simulink model "Ctrl_warning"  (R2018b)
settings: Solver=FixedStepDiscrete  StartTime=0.0  StopTime=10.0  FixedStep=0.1  RelTol=1e-3  EnableMultiTasking=on
values from neighbouring files (symbols this model uses):
  BASE_DATA_TYPE = mpt.Parameter    [warnings_interface_dd.m]
  EXTD_PAYLOAD_AVBLSTS = mpt.Parameter    [warnings_interface_dd.m]
  MASTER_LAMP_MASK = mpt.Parameter    [warnings_interface_dd.m]
  RED = mpt.Parameter    [warnings_interface_dd.m]
  WARN_ATTRIBUTES_ARRAY = mpt.Parameter    [Ctrl_warning_config.m]
  WARN_LAMP_CONFIGURED = mpt.Parameter    [Ctrl_warning_config.m]
  WRN_PAYLOAD_INITVAL = mpt.Parameter    [warnings_interface_dd.m]
  YELLOW = mpt.Parameter    [warnings_interface_dd.m]
undefined symbols (not defined in the file or in its folder): ExtWarningCurrentEvent, ExtWarningCurrentPayload, ExtWarningCurrentStatus, TotalNumOfWarnings, UI_WARNING_EVENT_FORCED, UI_WARNING_EVENT_NONE, UI_WARNING_EVENT_RETRIGGER, UI_WARNING_STATUS_OFF, UI_WARNING_STATUS_ON, WRNG_NOTIFIED_NONE, WRNG_NOTIFIED_SHOW
libraries: simulink x31, hdlsllib x3
settings Model: Creator=VRK  LastModifiedBy=VRK
settings DataIOCC: SaveOutput=off
settings OptimizationCC: DefaultParameterBehavior=Inlined  EnhancedBackFolding=on  PassReuseOutputArgsAs=Individual arguments  ZeroExternalMemoryAtStartup=off  ZeroInternalMemoryAtStartup=off  MaxStackSize=750  OptimizeBlockOrder=speed  DifferentSizesBufferReuse=on  OptimizationCustomize=off
settings DebuggingCC: ParameterTunabilityLossMsg=error
settings SFSimCC: MATLABDynamicMemAlloc=off
settings RTWCC: SystemTargetFile=autosar.tlc  GenCodeOnly=on  TemplateMakefile=ert_default_tmf  Description=AUTOSAR  GenerateReport=on  IncludeHyperlinkInReport=on  LaunchReport=on  PortableWordSizes=on  GenerateTraceInfo=on  GenerateTraceReport=on  GenerateTraceReportSl=on  GenerateTraceReportSf=on  GenerateTraceReportEml=on
settings CodeAppCC: ForceParamTrailComments=on  IgnoreCustomStorageClasses=off  OperatorAnnotations=on  SimulinkDataObjDesc=on  SFDataObjDesc=on  InsertBlockDesc=on
settings STFCustomTargetCC: TargetLangStandard=C99 (ISO)  MultiwordLength=256  ParMdlRefBuildCompliant=on  CompOptLevelCompliant=on  IncludeMdlTerminateFcn=off  CombineOutputUpdateFcns=on  SuppressErrorStatus=on  ERTCustomFileBanners=on  SupportNonFinite=off  SupportComplex=off  SupportContinuousTime=off  SupportNonInlinedSFcns=off  RemoveResetFunc=on  ParenthesesLevel=Maximum  CastingMode=Standards  MATLABClassNameForMDSCustomization=Simulink.SoftwareTarget.ERTCustomization  AutosarCompliant=on  UseToolchainInfoCompliant=on  LookupTableObjectStructAxisOrder=2,1,3,4,...  LUTObjectStructOrderEvenSpacing=Size,Table,Breakpoints  SystemTargetFile=autosar.tlc
settings ERTTargetCC: TargetLangStandard=C99 (ISO)  ConcurrentExecutionCompliant=off  IncludeMdlTerminateFcn=off  SuppressErrorStatus=on  SupportNonFinite=off  SupportComplex=off  ParenthesesLevel=Maximum  CastingMode=Standards  ModelStepFunctionPrototypeControlCompliant=off  CPPClassGenCompliant=off  AutosarCompliant=on  LookupTableObjectStructAxisOrder=2,1,3,4,...  LUTObjectStructOrderEvenSpacing=Size,Table,Breakpoints  InlinedParameterPlacement=NonHierarchical  ERTCustomFileTemplate=example_file_process.tlc  ERTFilePackagingFormat=CompactWithDataFile

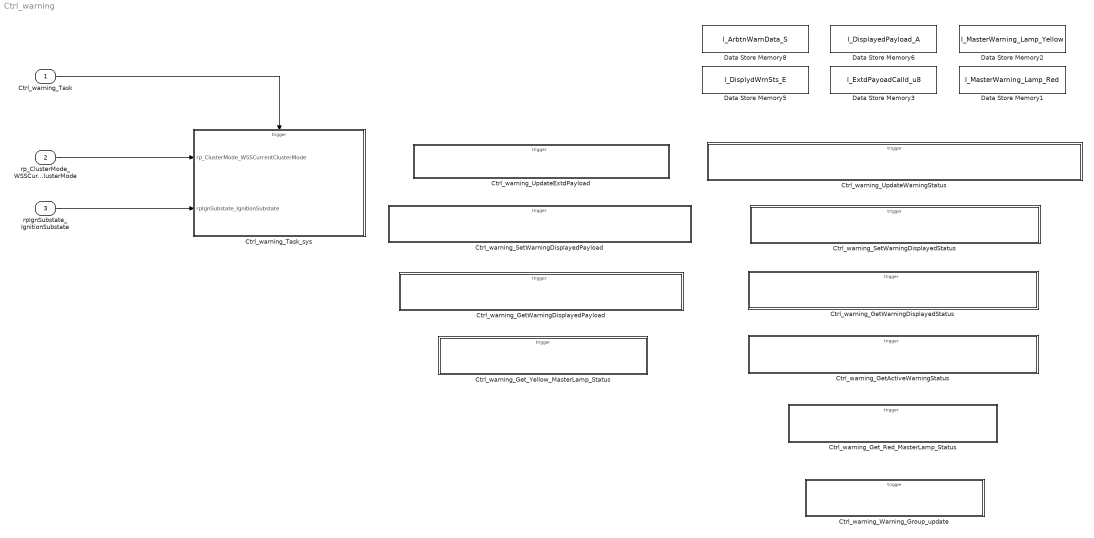
== system Ctrl_warning ==
  Ctrl_warning_Task : Inport  SampleTime=0.1  OutputFunctionCall=on
  rp_ClusterMode_WSSCurrentClusterMode : Inport  Port=2  OutDataTypeStr=ClusterModes  PortDimensions=1
  rpIgnSubstate_IgnitionSubstate : Inport  Port=3  OutDataTypeStr=IgntionSubstateType  PortDimensions=1
  Ctrl_warning_GetActiveWarningStatus : Subsystem  TreatAsAtomicUnit=on
  Ctrl_warning_GetWarningDisplayedPayload : Subsystem  TreatAsAtomicUnit=on
  Ctrl_warning_GetWarningDisplayedStatus : Subsystem  TreatAsAtomicUnit=on
  Ctrl_warning_Get_Red_MasterLamp_Status : Subsystem  TreatAsAtomicUnit=on
  Ctrl_warning_Get_Yellow_MasterLamp_Status : Subsystem  TreatAsAtomicUnit=on
  Ctrl_warning_SetWarningDisplayedPayload : Subsystem  TreatAsAtomicUnit=on
  Ctrl_warning_SetWarningDisplayedStatus : Subsystem  TreatAsAtomicUnit=on
  Ctrl_warning_Task_sys : Subsystem  TreatAsAtomicUnit=on
  Ctrl_warning_UpdateExtdPayload : Subsystem  TreatAsAtomicUnit=on
  Ctrl_warning_UpdateWarningStatus : Subsystem  TreatAsAtomicUnit=on
  Ctrl_warning_Warning_Group_update : Subsystem  TreatAsAtomicUnit=on
  Data Store Memory1 : DataStoreMemory  DataStoreName=l_MasterWarning_Lamp_Red  ReadBeforeWriteMsg=warning  WriteAfterWriteMsg=warning  WriteAfterReadMsg=warning  VectorParams1D=off  ShowAdditionalParam=off  OutDataTypeStr=uint8  Dimensions=14
  Data Store Memory2 : DataStoreMemory  DataStoreName=l_MasterWarning_Lamp_Yellow  ReadBeforeWriteMsg=warning  WriteAfterWriteMsg=warning  WriteAfterReadMsg=warning  VectorParams1D=off  ShowAdditionalParam=off  OutDataTypeStr=uint8  Dimensions=14
  Data Store Memory3 : DataStoreMemory  DataStoreName=l_ExtdPayoadCalld_u8  ReadBeforeWriteMsg=warning  WriteAfterWriteMsg=warning  WriteAfterReadMsg=warning  InitialValue=zeros(1,560)  VectorParams1D=off  ShowAdditionalParam=off  OutDataTypeStr=uint8
  Data Store Memory5 : DataStoreMemory  DataStoreName=l_DisplydWrnSts_E  ReadBeforeWriteMsg=warning  WriteAfterWriteMsg=warning  WriteAfterReadMsg=warning  VectorParams1D=off  ShowAdditionalParam=off  OutDataTypeStr=WarningDisplayedStatus  Dimensions=14
  Data Store Memory6 : DataStoreMemory  DataStoreName=l_DisplayedPayload_A  ReadBeforeWriteMsg=warning  WriteAfterWriteMsg=warning  WriteAfterReadMsg=warning  InitialValue=zeros(1,602)  ShowAdditionalParam=off  OutDataTypeStr=Bus: WarningPayload_Type
  Data Store Memory8 : DataStoreMemory  DataStoreName=l_ArbtnWarnData_S  ReadBeforeWriteMsg=warning  WriteAfterWriteMsg=warning  WriteAfterReadMsg=warning  InitialValue=zeros(1,560)  VectorParams1D=off  ShowAdditionalParam=off  OutDataTypeStr=Bus:ExtWarningData
  wires:
  Ctrl_warning_Task/1 -> Ctrl_warning_Task_sys/Trigger
  rp_ClusterMode_WSSCurrentClusterMode/1 -> Ctrl_warning_Task_sys/1(rp_ClusterMode_WSSCurrentClusterMode)
  rpIgnSubstate_IgnitionSubstate/1 -> Ctrl_warning_Task_sys/2(rpIgnSubstate_IgnitionSubstate)

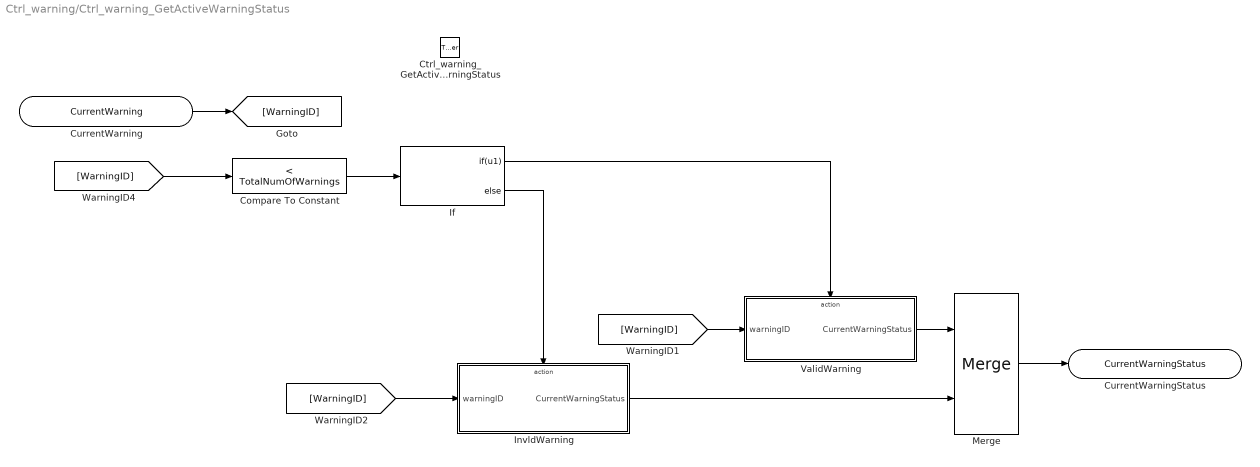
== system Ctrl_warning/Ctrl_warning_GetActiveWarningStatus ==
  Ctrl_warning_GetActiveWarningStatus : TriggerPort  TriggerType=function-call  IsSimulinkFunction=on  FunctionName=Ctrl_warning_GetActiveWarningStatus  VariantControl=(inherit)
  Compare To Constant : simulink/Logic and Bit Operations/Compare To Constant  relop=<  const=TotalNumOfWarnings  OutDataTypeStr=boolean
  If : If  IfExpression=u1
  InvldWarning : Subsystem
  Merge : Merge
  ValidWarning : Subsystem
  CurrentWarning : ArgIn  DisableCoverage=on  OutDataTypeStr=WarningId  ArgumentName=CurrentWarning
  CurrentWarningStatus : ArgOut  DisableCoverage=on  OutDataTypeStr=Bus:ExtWarningData  ArgumentName=CurrentWarningStatus
  wires:
  Compare To Constant/1 -> If/1
  [WarningID] -> ValidWarning/1(warningID)
  ValidWarning/1(CurrentWarningStatus) -> Merge/1
  If/2 -> InvldWarning/Action
  [WarningID] -> InvldWarning/1(warningID)
  If/1 -> ValidWarning/Action
  InvldWarning/1(CurrentWarningStatus) -> Merge/2
  [WarningID] -> Compare To Constant/1
  CurrentWarning/1 -> [WarningID]
  Merge/1 -> CurrentWarningStatus/1

== system Ctrl_warning/Ctrl_warning_GetWarningDisplayedPayload ==
  Ctrl_warning_GetWarningDisplayedPayload : TriggerPort  TriggerType=function-call  IsSimulinkFunction=on  FunctionName=Ctrl_warning_GetWarningDisplayedPayload  VariantControl=(inherit)
  Compare To Constant1 : simulink/Logic and Bit Operations/Compare To Constant  relop=<  const=TotalNumOfWarnings  OutDataTypeStr=boolean
  If : If  IfExpression=u1  ShowElse=off
  ValidWarnInvoked : Subsystem  TreatAsAtomicUnit=on
  CurWarningId : ArgIn  DisableCoverage=on  OutDataTypeStr=WarningId  ArgumentName=CurWarningId
  DisplayedPayload : ArgOut  DisableCoverage=on  OutDataTypeStr=PayloadArr_u8_8  PortDimensions=8  ArgumentName=DisplayedPayload
  wires:
  CurWarningId/1 -> ValidWarnInvoked/1(WarningId), Compare To Constant1/1
  If/1 -> ValidWarnInvoked/Action
  Compare To Constant1/1 -> If/1
  ValidWarnInvoked/1(DispdPayload) -> DisplayedPayload/1

== system Ctrl_warning/Ctrl_warning_GetWarningDisplayedStatus ==
  Ctrl_warning_GetWarningDisplayedStatus : TriggerPort  TriggerType=function-call  IsSimulinkFunction=on  FunctionName=Ctrl_warning_GetWarningDisplayedStatus  VariantControl=(inherit)
  Compare To Constant : simulink/Logic and Bit Operations/Compare To Constant  relop=<  const=TotalNumOfWarnings  OutDataTypeStr=boolean
  Constant1 : Constant  Value=WRNG_NOTIFIED_NONE  OutDataTypeStr=uint8
  Data Store Read : DataStoreRead  DataStoreName=l_DisplydWrnSts_E
  Selector : Selector  IndexMode=Zero-based  IndexOptions=Index vector (port)  Indices=[1 3]  OutputSizes=1
  Switch : Switch  Criteria=u2 ~= 0
  CurWarningId : ArgIn  DisableCoverage=on  OutDataTypeStr=WarningId  ArgumentName=CurWarningId
  DisplayedStatus : ArgOut  DisableCoverage=on  OutDataTypeStr=WarningDisplayedStatus  ArgumentName=DisplayedStatus
  wires:
  Selector/1 -> Switch/1
  Constant1/1 -> Switch/3
  Compare To Constant/1 -> Switch/2
  Data Store Read/1 -> Selector/1
  CurWarningId/1 -> Selector/2, Compare To Constant/1
  Switch/1 -> DisplayedStatus/1

== system Ctrl_warning/Ctrl_warning_Get_Red_MasterLamp_Status ==
  Ctrl_warning_Get_Red_MasterLamp_Status : TriggerPort  TriggerType=function-call  IsSimulinkFunction=on  FunctionName=Ctrl_warning_Get_Red_MasterLamp_Status  VariantControl=(inherit)
  Chart : Stateflow chart  TreatAsAtomicUnit=on
  LampStatus : ArgOut  DisableCoverage=on  OutDataTypeStr=uint8  ArgumentName=LampStatus
  wires:
  Chart/1(fl_RedLampSts_u8) -> LampStatus/1

== system Ctrl_warning/Ctrl_warning_Get_Yellow_MasterLamp_Status ==
  Ctrl_warning_Get_Yellow_MasterLamp_Status : TriggerPort  TriggerType=function-call  IsSimulinkFunction=on  FunctionName=Ctrl_warning_Get_Yellow_MasterLamp_Status  VariantControl=(inherit)
  Chart : Stateflow chart  TreatAsAtomicUnit=on
  LampStatus : ArgOut  DisableCoverage=on  OutDataTypeStr=uint8  ArgumentName=LampStatus
  wires:
  Chart/1(fl_YellowLampSts_u8) -> LampStatus/1

== system Ctrl_warning/Ctrl_warning_SetWarningDisplayedPayload ==
  Ctrl_warning_SetWarningDisplayedPayload : TriggerPort  TriggerType=function-call  IsSimulinkFunction=on  FunctionName=Ctrl_warning_SetWarningDisplayedPayload  VariantControl=(inherit)
  Compare To Constant : simulink/Logic and Bit Operations/Compare To Constant  relop=<  const=TotalNumOfWarnings  OutDataTypeStr=boolean
  If : If  IfExpression=u1  ShowElse=off
  ValidPayload : Subsystem  TreatAsAtomicUnit=on
  CurWarningId : ArgIn  DisableCoverage=on  OutDataTypeStr=WarningId  ArgumentName=CurWarningId
  CurWarningDispPayload : ArgIn  Port=2  OutDataTypeStr=uint8  PortDimensions=8  ArgumentName=CurWarningDispPayload
  wires:
  CurWarningId/1 -> ValidPayload/1(WarningId), Compare To Constant/1
  Compare To Constant/1 -> If/1
  If/1 -> ValidPayload/Action
  CurWarningDispPayload/1 -> ValidPayload/2(Payload)

== system Ctrl_warning/Ctrl_warning_SetWarningDisplayedStatus ==
  Ctrl_warning_SetWarningDisplayedStatus : TriggerPort  TriggerType=function-call  IsSimulinkFunction=on  FunctionName=Ctrl_warning_SetWarningDisplayedStatus  VariantControl=(inherit)
  Compare To Constant : simulink/Logic and Bit Operations/Compare To Constant  relop=<  const=TotalNumOfWarnings  OutDataTypeStr=boolean
  If : If  IfExpression=u1  ShowElse=off
  StatusofValidWarningID : Subsystem
  CurWarningId : ArgIn  DisableCoverage=on  OutDataTypeStr=WarningId  ArgumentName=CurWarningId
  CurWarningDispStatus : ArgIn  Port=2  OutDataTypeStr=WarningDisplayedStatus  ArgumentName=CurWarningDispStatus
  wires:
  If/1 -> StatusofValidWarningID/Action
  CurWarningId/1 -> StatusofValidWarningID/1(warningID), Compare To Constant/1
  Compare To Constant/1 -> If/1
  CurWarningDispStatus/1 -> StatusofValidWarningID/2(WarningStatus)

== system Ctrl_warning/Ctrl_warning_Task_sys ==
  rp_ClusterMode_WSSCurrentClusterMode : Inport  OutDataTypeStr=ClusterModes  PortDimensions=1
  rpIgnSubstate_IgnitionSubstate : Inport  Port=2  OutDataTypeStr=IgntionSubstateType  PortDimensions=1
  function : TriggerPort  TriggerType=function-call  VariantControl=Variant  SampleTimeType=periodic  SampleTime=-1
  InputHarness : Subsystem  Variant=on
  Terminator : Terminator
  Terminator1 : Terminator
  wires:
  rp_ClusterMode_WSSCurrentClusterMode/1 -> InputHarness/1(rp_ClusterMode_WSSCurrentClusterMode)
  rpIgnSubstate_IgnitionSubstate/1 -> InputHarness/2(rpIgnSubstate_IgnitionSubstate)
  InputHarness/1(rp_ClusterMode_WSSCurrentClusterMode_out) -> Terminator/1
  InputHarness/2(rpIgnSubstate_IgnitionSubstate_out) -> Terminator1/1

== system Ctrl_warning/Ctrl_warning_UpdateExtdPayload ==
  Ctrl_warning_UpdateExtdPayload : TriggerPort  TriggerType=function-call  IsSimulinkFunction=on  FunctionName=Ctrl_warning_UpdateExtdPayload  VariantControl=(inherit)
  Compare To Constant : simulink/Logic and Bit Operations/Compare To Constant  relop=<  const=TotalNumOfWarnings  OutDataTypeStr=boolean
  If : If  IfExpression=u1  ShowElse=off
  VldWarnId : Subsystem  TreatAsAtomicUnit=on
  WarningCurId : ArgIn  DisableCoverage=on  OutDataTypeStr=WarningId  ArgumentName=WarningCurId
  WarningPayload : ArgIn  Port=2  OutDataTypeStr=uint8  PortDimensions=8  ArgumentName=WarningPayload
  wires:
  WarningCurId/1 -> VldWarnId/1(WarningCurId), Compare To Constant/1
  Compare To Constant/1 -> If/1
  If/1 -> VldWarnId/Action
  WarningPayload/1 -> VldWarnId/2(WarningPayload)

== system Ctrl_warning/Ctrl_warning_UpdateWarningStatus ==
  Ctrl_warning_UpdateWarningStatus : TriggerPort  TriggerType=function-call  IsSimulinkFunction=on  FunctionName=Ctrl_warning_UpdateWarningStatus  VariantControl=(inherit)
  Compare To Constant : simulink/Logic and Bit Operations/Compare To Constant  relop=<  const=TotalNumOfWarnings  OutDataTypeStr=boolean
  If : If  IfExpression=u1  ShowElse=off
  UpdateWarningProperties : Subsystem
  WarningCurId : ArgIn  DisableCoverage=on  OutDataTypeStr=WarningId  ArgumentName=WarningCurId
  WarningCurStatus : ArgIn  Port=2  OutDataTypeStr=WarningStatus  ArgumentName=WarningCurStatus
  WarningCurEvent : ArgIn  Port=3  OutDataTypeStr=WarningEvent  ArgumentName=WarningCurEvent
  WarningPayload : ArgIn  Port=4  OutDataTypeStr=uint32  ArgumentName=WarningPayload
  wires:
  Compare To Constant/1 -> If/1
  If/1 -> UpdateWarningProperties/Action
  WarningCurId/1 -> UpdateWarningProperties/1(warningID), Compare To Constant/1
  WarningCurStatus/1 -> UpdateWarningProperties/2(WarningStatus)
  WarningCurEvent/1 -> UpdateWarningProperties/3(EventType)
  WarningPayload/1 -> UpdateWarningProperties/4(PayloadValue)

== system Ctrl_warning/Ctrl_warning_Warning_Group_update ==
  Ctrl_warning_Warning_Group_update : TriggerPort  TriggerType=function-call  IsSimulinkFunction=on  FunctionName=Ctrl_warning_Warning_Group_update  VariantControl=(inherit)

== system Ctrl_warning/Ctrl_warning_GetActiveWarningStatus/InvldWarning ==
  warningID : Inport
  Action Port : ActionPort  ActionType=else
  Bus Assignment : BusAssignment  AssignedSignals=ExtWarningCurrentStatus,ExtWarningCurrentEvent,ExtWarningCurrentPayload
  Constant : Constant  Value=zeros(1,8)  OutDataTypeStr=PayloadArr_u8_8
  Constant1 : Constant  Value=UI_WARNING_STATUS_OFF  OutDataTypeStr=uint8
  Constant3 : Constant  Value=UI_WARNING_EVENT_NONE  OutDataTypeStr=uint8
  Data Store Read : DataStoreRead  DataStoreName=l_ArbtnWarnData_S
  Selector : Selector  IndexMode=Zero-based  IndexOptions=Index vector (port)  Indices=[1 3]  OutputSizes=1
  CurrentWarningStatus : Outport
  wires:
  Data Store Read/1 -> Selector/1
  warningID/1 -> Selector/2
  Constant1/1 -> Bus Assignment/2
  Constant3/1 -> Bus Assignment/3
  Bus Assignment/1 -> CurrentWarningStatus/1
  Selector/1 -> Bus Assignment/1
  Constant/1 -> Bus Assignment/4

== system Ctrl_warning/Ctrl_warning_GetActiveWarningStatus/ValidWarning ==
  warningID : Inport
  Action Port : ActionPort  ActionType=then
  Data Store Read : DataStoreRead  DataStoreName=l_ArbtnWarnData_S
  Selector : Selector  IndexMode=Zero-based  IndexOptions=Index vector (port)  Indices=[1 3]  OutputSizes=1
  CurrentWarningStatus : Outport
  wires:
  warningID/1 -> Selector/2
  Data Store Read/1 -> Selector/1
  Selector/1 -> CurrentWarningStatus/1

== system Ctrl_warning/Ctrl_warning_GetWarningDisplayedPayload/ValidWarnInvoked ==
  WarningId : Inport
  Action Port : ActionPort  ActionType=then
  Bus Selector : BusSelector  OutputSignals=WarningPayloadRecd
  Data Store Read2 : DataStoreRead  DataStoreName=l_DisplayedPayload_A
  Selector1 : Selector  IndexMode=Zero-based  IndexOptions=Index vector (port)  Indices=[1 3]  OutputSizes=1
  DispdPayload : Outport  PortDimensions=8
  wires:
  WarningId/1 -> Selector1/2
  Bus Selector/1 -> DispdPayload/1  "<WarningPayloadRecd>"
  Data Store Read2/1 -> Selector1/1
  Selector1/1 -> Bus Selector/1

== system Ctrl_warning/Ctrl_warning_SetWarningDisplayedPayload/ValidPayload ==
  WarningId : Inport  OutDataTypeStr=uint16
  Payload : Inport  Port=2  PortDimensions=8
  Action Port : ActionPort  ActionType=then
  Assignment1 : Assignment  IndexMode=Zero-based  DiagnosticForDimensions=Warning  IndexOptions=Index vector (port)  Indices=1  OutputSizes=1
  Bus Assignment : BusAssignment  AssignedSignals=WarningPayloadRecd
  Data Store Read : DataStoreRead  DataStoreName=l_DisplayedPayload_A
  Data Store Read9 : DataStoreRead  DataStoreName=l_DisplayedPayload_A
  Data Store Write : DataStoreWrite  DataStoreName=l_DisplayedPayload_A
  Selector1 : Selector  IndexMode=Zero-based  IndexOptions=Index vector (port)  Indices=[1 3]  OutputSizes=1
  wires:
  Data Store Read/1 -> Selector1/1
  Assignment1/1 -> Data Store Write/1
  WarningId/1 -> Assignment1/3, Selector1/2
  Payload/1 -> Bus Assignment/2
  Selector1/1 -> Bus Assignment/1
  Data Store Read9/1 -> Assignment1/1
  Bus Assignment/1 -> Assignment1/2

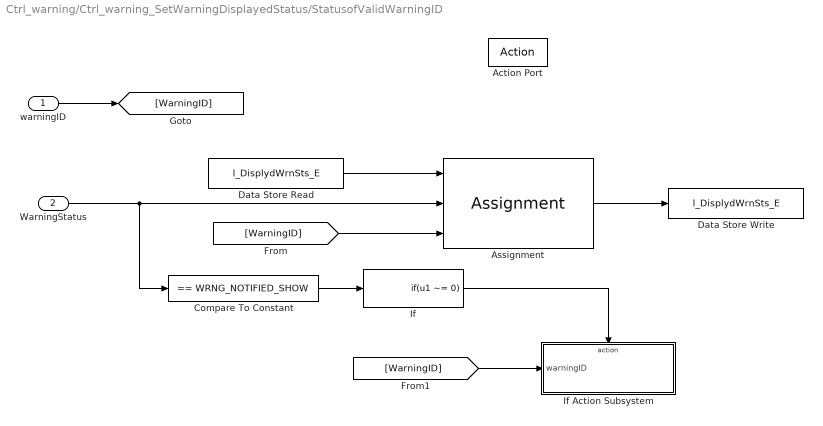
== system Ctrl_warning/Ctrl_warning_SetWarningDisplayedStatus/StatusofValidWarningID ==
  warningID : Inport
  WarningStatus : Inport  Port=2
  Action Port : ActionPort  ActionType=then
  Assignment : Assignment  IndexMode=Zero-based  DiagnosticForDimensions=Warning  IndexOptions=Index vector (port)  Indices=1  OutputSizes=14
  Compare To Constant : simulink/Logic and Bit Operations/Compare To Constant  relop===  const=WRNG_NOTIFIED_SHOW  OutDataTypeStr=boolean
  Data Store Read : DataStoreRead  DataStoreName=l_DisplydWrnSts_E
  Data Store Write : DataStoreWrite  DataStoreName=l_DisplydWrnSts_E
  If : If  IfExpression=u1 ~= 0  ShowElse=off
  If Action Subsystem : Subsystem  TreatAsAtomicUnit=on
  wires:
  Assignment/1 -> Data Store Write/1
  WarningStatus/1 -> Compare To Constant/1, Assignment/2
  Compare To Constant/1 -> If/1
  If/1 -> If Action Subsystem/Action
  warningID/1 -> [WarningID]
  [WarningID] -> If Action Subsystem/1(warningID)
  [WarningID] -> Assignment/3
  Data Store Read/1 -> Assignment/1

== system Ctrl_warning/Ctrl_warning_Task_sys/InputHarness ==
  rp_ClusterMode_WSSCurrentClusterMode : Inport  OutDataTypeStr=ClusterModes  PortDimensions=1
  rpIgnSubstate_IgnitionSubstate : Inport  Port=2  OutDataTypeStr=IgntionSubstateType  PortDimensions=1
  CodeGeneration : Subsystem  VariantControl=CODEGENERATION
  Simulation : Subsystem  VariantControl=SIMULATION
  rp_ClusterMode_WSSCurrentClusterMode_out : Outport  OutDataTypeStr=ClusterModes  PortDimensions=1
  rpIgnSubstate_IgnitionSubstate_out : Outport  Port=2  OutDataTypeStr=IgntionSubstateType  PortDimensions=1

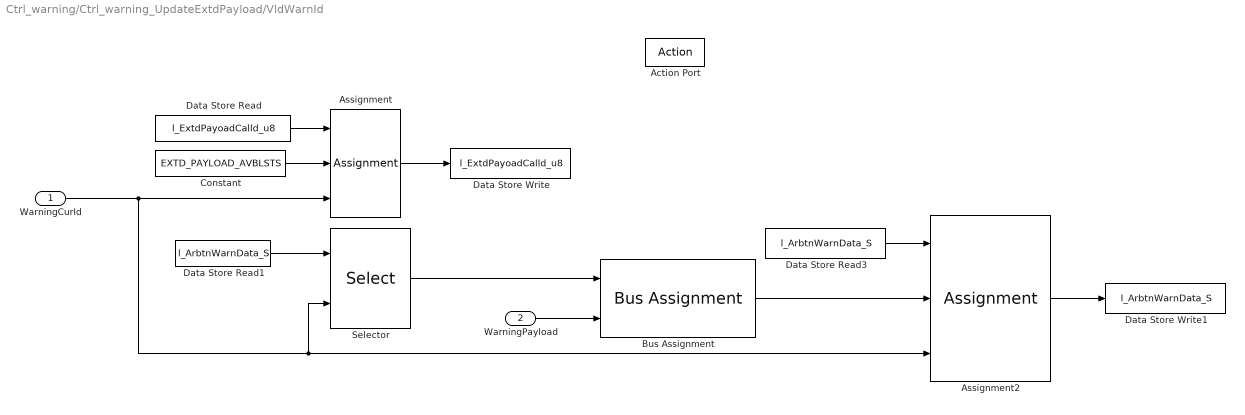
== system Ctrl_warning/Ctrl_warning_UpdateExtdPayload/VldWarnId ==
  WarningCurId : Inport
  WarningPayload : Inport  Port=2
  Action Port : ActionPort  ActionType=then
  Assignment : Assignment  IndexMode=Zero-based  DiagnosticForDimensions=Warning  IndexOptions=Index vector (port)  Indices=1  OutputSizes=1
  Assignment2 : Assignment  IndexMode=Zero-based  DiagnosticForDimensions=Warning  IndexOptions=Index vector (port)  Indices=1  OutputSizes=14
  Bus Assignment : BusAssignment  AssignedSignals=ExtWarningCurrentPayload
  Constant : Constant  Value=EXTD_PAYLOAD_AVBLSTS
  Data Store Read : DataStoreRead  DataStoreName=l_ExtdPayoadCalld_u8
  Data Store Read1 : DataStoreRead  DataStoreName=l_ArbtnWarnData_S
  Data Store Read3 : DataStoreRead  DataStoreName=l_ArbtnWarnData_S
  Data Store Write : DataStoreWrite  DataStoreName=l_ExtdPayoadCalld_u8
  Data Store Write1 : DataStoreWrite  DataStoreName=l_ArbtnWarnData_S
  Selector : Selector  IndexMode=Zero-based  IndexOptions=Index vector (port)  Indices=[1 3]  OutputSizes=1
  wires:
  Data Store Read/1 -> Assignment/1
  Assignment/1 -> Data Store Write/1
  WarningCurId/1 -> Selector/2, Assignment2/3, Assignment/3
  Constant/1 -> Assignment/2
  Selector/1 -> Bus Assignment/1
  Data Store Read3/1 -> Assignment2/1
  Bus Assignment/1 -> Assignment2/2
  Assignment2/1 -> Data Store Write1/1
  Data Store Read1/1 -> Selector/1
  WarningPayload/1 -> Bus Assignment/2

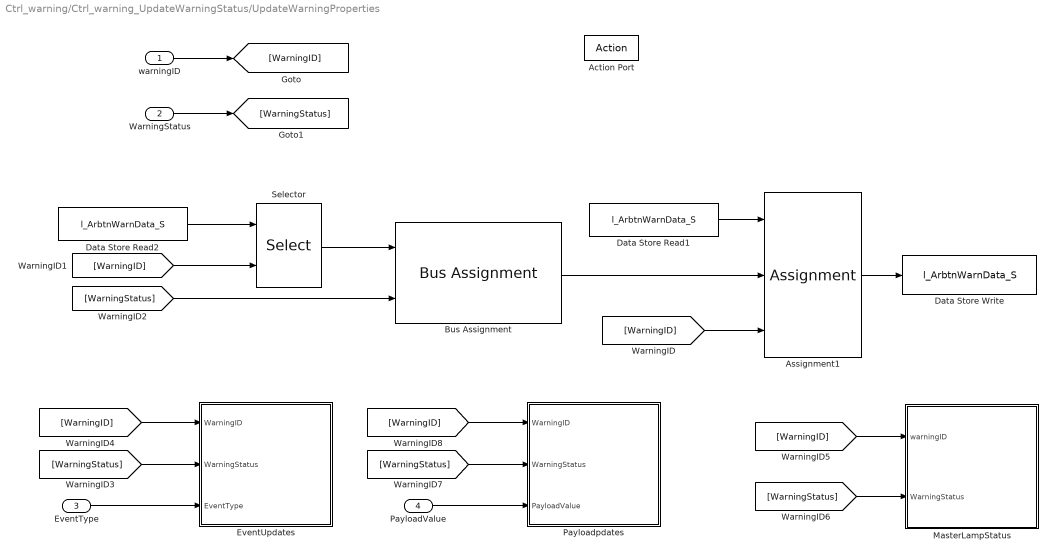
== system Ctrl_warning/Ctrl_warning_UpdateWarningStatus/UpdateWarningProperties ==
  warningID : Inport
  WarningStatus : Inport  Port=2
  EventType : Inport  Port=3
  PayloadValue : Inport  Port=4  OutDataTypeStr=uint32
  Action Port : ActionPort  ActionType=then
  Assignment1 : Assignment  IndexMode=Zero-based  DiagnosticForDimensions=Warning  IndexOptions=Index vector (port)  Indices=1  OutputSizes=14
  Bus Assignment : BusAssignment  AssignedSignals=ExtWarningCurrentStatus
  Data Store Read1 : DataStoreRead  DataStoreName=l_ArbtnWarnData_S
  Data Store Read2 : DataStoreRead  DataStoreName=l_ArbtnWarnData_S
  Data Store Write : DataStoreWrite  DialogController=Simulink.DDGSource  DataStoreName=l_ArbtnWarnData_S
  EventUpdates : Subsystem  TreatAsAtomicUnit=on
      settings: RTWSystemCode=Inline
  MasterLampStatus : Subsystem  TreatAsAtomicUnit=on  RTWFcnName=update_MasterWarning_Lamp
      settings: RTWSystemCode=Nonreusable function  RTWFcnNameOpts=User specified
  Payloadpdates : Subsystem  TreatAsAtomicUnit=on
      settings: RTWSystemCode=Inline
  Selector : Selector  IndexMode=Zero-based  IndexOptions=Index vector (port)  Indices=[1 3]  OutputSizes=1
  wires:
  Selector/1 -> Bus Assignment/1
  Bus Assignment/1 -> Assignment1/2
  Assignment1/1 -> Data Store Write/1
  PayloadValue/1 -> Payloadpdates/3(PayloadValue)
  warningID/1 -> [WarningID]
  [WarningID] -> Selector/2
  [WarningID] -> Assignment1/3
  [WarningID] -> MasterLampStatus/1(warningID)
  [WarningStatus] -> MasterLampStatus/2(WarningStatus)
  WarningStatus/1 -> [WarningStatus]
  [WarningStatus] -> Bus Assignment/2
  [WarningStatus] -> EventUpdates/2(WarningStatus)
  [WarningID] -> EventUpdates/1("WarningID ")
  EventType/1 -> EventUpdates/3(EventType)
  Data Store Read1/1 -> Assignment1/1
  Data Store Read2/1 -> Selector/1
  [WarningStatus] -> Payloadpdates/2(WarningStatus)
  [WarningID] -> Payloadpdates/1("WarningID ")

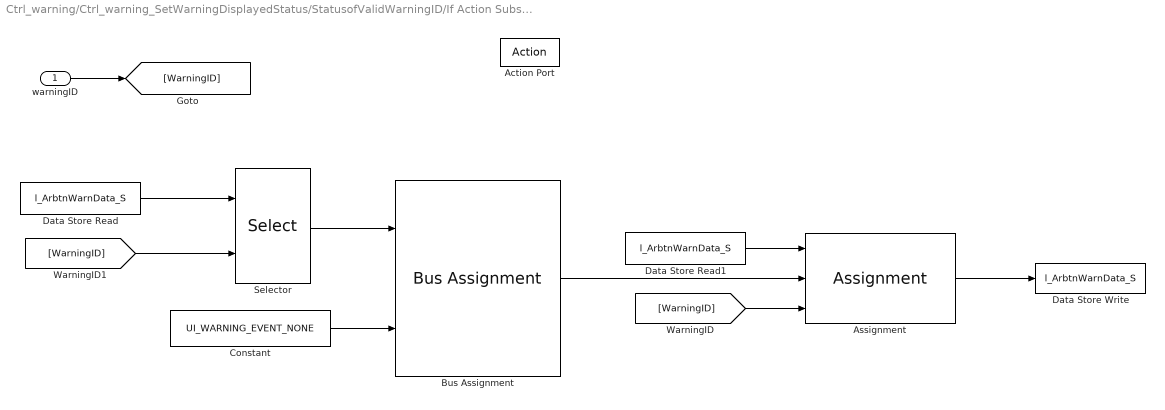
== system Ctrl_warning/Ctrl_warning_SetWarningDisplayedStatus/StatusofValidWarningID/If Action Subsystem ==
  warningID : Inport
  Action Port : ActionPort  ActionType=then
  Assignment : Assignment  IndexMode=Zero-based  IndexOptions=Index vector (port)  Indices=1  OutputSizes=14
  Bus Assignment : BusAssignment  AssignedSignals=ExtWarningCurrentEvent
  Constant : Constant  Value=UI_WARNING_EVENT_NONE  OutDataTypeStr=uint8
  Data Store Read : DataStoreRead  DataStoreName=l_ArbtnWarnData_S
  Data Store Read1 : DataStoreRead  DataStoreName=l_ArbtnWarnData_S
  Data Store Write : DataStoreWrite  DataStoreName=l_ArbtnWarnData_S
  Selector : Selector  IndexMode=Zero-based  IndexOptions=Index vector (port)  Indices=[1 3]  OutputSizes=1
  wires:
  Bus Assignment/1 -> Assignment/2
  Assignment/1 -> Data Store Write/1
  [WarningID] -> Assignment/3
  warningID/1 -> [WarningID]
  Constant/1 -> Bus Assignment/2
  [WarningID] -> Selector/2
  Data Store Read/1 -> Selector/1
  Selector/1 -> Bus Assignment/1
  Data Store Read1/1 -> Assignment/1

== system Ctrl_warning/Ctrl_warning_Task_sys/InputHarness/CodeGeneration ==
  rp_ClusterMode_WSSCurrentClusterMode : Inport  OutDataTypeStr=ClusterModes  PortDimensions=1
  rpIgnSubstate_IgnitionSubstate : Inport  Port=2  OutDataTypeStr=IgntionSubstateType  PortDimensions=1
  rp_ClusterMode_WSSCurrentClusterMode_out : Outport  OutDataTypeStr=ClusterModes  PortDimensions=1
  rpIgnSubstate_IgnitionSubstate_out : Outport  Port=2  OutDataTypeStr=IgntionSubstateType  PortDimensions=1
  wires:
  rp_ClusterMode_WSSCurrentClusterMode/1 -> rp_ClusterMode_WSSCurrentClusterMode_out/1
  rpIgnSubstate_IgnitionSubstate/1 -> rpIgnSubstate_IgnitionSubstate_out/1

== system Ctrl_warning/Ctrl_warning_Task_sys/InputHarness/Simulation ==

== system Ctrl_warning/Ctrl_warning_UpdateWarningStatus/UpdateWarningProperties/EventUpdates ==
  "WarningID " : Inport
  WarningStatus : Inport  Port=2
  EventType : Inport  Port=3
  Compare To Constant : simulink/Logic and Bit Operations/Compare To Constant  relop===  const=UI_WARNING_STATUS_OFF  OutDataTypeStr=boolean
  EventNone : Subsystem  TreatAsAtomicUnit=on
      settings: RTWSystemCode=Inline
  EventUpdate : Subsystem  TreatAsAtomicUnit=on
      settings: RTWSystemCode=Inline
  If : If  IfExpression=u1 ~= 0
  wires:
  WarningStatus/1 -> Compare To Constant/1
  Compare To Constant/1 -> If/1
  If/1 -> EventNone/Action
  If/2 -> EventUpdate/Action
  "WarningID "/1 -> EventNone/1("WarningID "), EventUpdate/1(WarningID)
  EventType/1 -> EventUpdate/2(EventType)

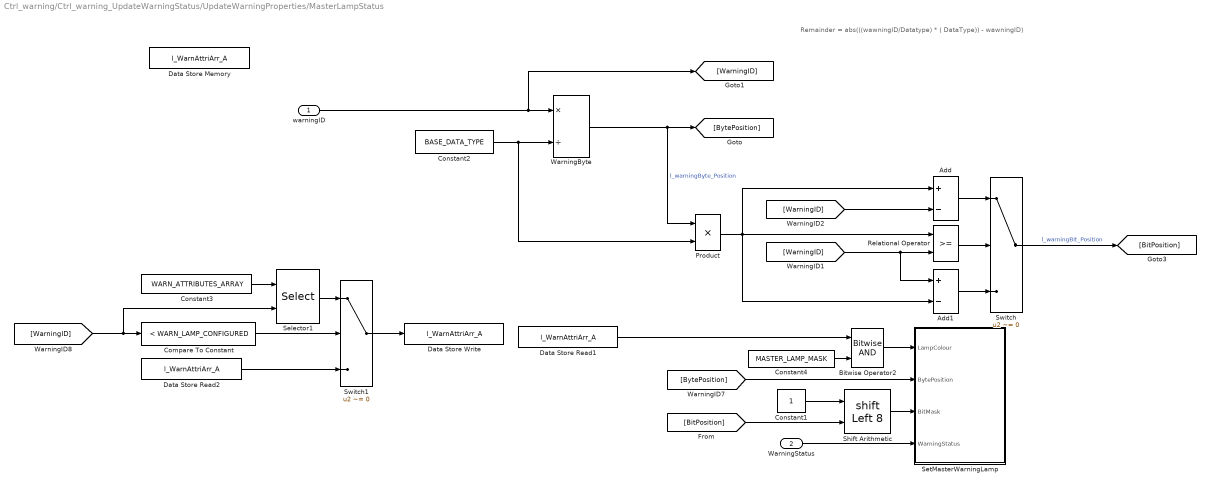
== system Ctrl_warning/Ctrl_warning_UpdateWarningStatus/UpdateWarningProperties/MasterLampStatus ==
  note: Remainder = abs(((wawningID/Datatype) * ( DataType)) - wawningID)
  warningID : Inport  OutDataTypeStr=uint16
  WarningStatus : Inport  Port=2  OutDataTypeStr=uint8
  Add : Sum  Inputs=+-
  Add1 : Sum  Inputs=+-
  Bitwise Operator2 : simulink/Logic and Bit Operations/Bitwise Operator  logicop=AND  UseBitMask=off  NumInputPorts=2  BitMask=bin2dec('11011001')  BitMaskRealWorld=Stored Integer
  Compare To Constant : simulink/Logic and Bit Operations/Compare To Constant  relop=<  const=WARN_LAMP_CONFIGURED  OutDataTypeStr=boolean
  Constant1 : Constant  OutDataTypeStr=uint8
  Constant2 : Constant  Value=BASE_DATA_TYPE
  Constant3 : Constant  Value=WARN_ATTRIBUTES_ARRAY  OutDataTypeStr=uint8
  Constant4 : Constant  Value=MASTER_LAMP_MASK  OutDataTypeStr=uint8
  Data Store Memory : DataStoreMemory  DataStoreName=l_WarnAttriArr_A  ReadBeforeWriteMsg=warning  WriteAfterWriteMsg=warning  WriteAfterReadMsg=warning  ShowAdditionalParam=off  OutDataTypeStr=uint8
  Data Store Read1 : DataStoreRead  DataStoreName=l_WarnAttriArr_A
  Data Store Read2 : DataStoreRead  DataStoreName=l_WarnAttriArr_A
  Data Store Write : DataStoreWrite  DataStoreName=l_WarnAttriArr_A
  Product : Product  OutDataTypeStr=uint16  RndMeth=Zero
  Relational Operator : RelationalOperator  OutDataTypeStr=boolean  RndMeth=Nearest
  Selector1 : Selector  IndexMode=Zero-based  IndexOptions=Index vector (port)  Indices=[1 3]  OutputSizes=1
  SetMasterWarningLamp : Subsystem  TreatAsAtomicUnit=on
  Shift Arithmetic : ArithShift  BitShiftNumberSource=Input port  BitShiftNumber=8  BitShiftDirection=Left  DiagnosticForOORShift=Error
      settings: InputPortMap=u0,p1
  Switch : Switch  Criteria=u2 ~= 0  RndMeth=Zero
  Switch1 : Switch  Criteria=u2 ~= 0  OutDataTypeStr=uint8  RndMeth=Zero
  WarningByte : Product  Inputs=*/  OutDataTypeStr=uint16  RndMeth=Zero
  wires:
  warningID/1 -> [WarningID], WarningByte/1
  WarningByte/1 -> Product/1, [BytePosition]  "l_warningByte_Position"
  [WarningID] -> Add/2
  [WarningID] -> Add1/1, Relational Operator/2
  Product/1 -> Add/1, Add1/2, Relational Operator/1
  Add/1 -> Switch/1
  Relational Operator/1 -> Switch/2
  Add1/1 -> Switch/3
  Switch/1 -> [BitPosition]  "l_warningBit_Position"
  Constant1/1 -> Shift Arithmetic/1
  [BitPosition] -> Shift Arithmetic/2
  Bitwise Operator2/1 -> SetMasterWarningLamp/1(LampColour)
  Shift Arithmetic/1 -> SetMasterWarningLamp/3(BitMask)
  [BytePosition] -> SetMasterWarningLamp/2(BytePosition)
  WarningStatus/1 -> SetMasterWarningLamp/4(WarningStatus)
  Constant3/1 -> Selector1/1
  Constant4/1 -> Bitwise Operator2/2
  Compare To Constant/1 -> Switch1/2
  [WarningID] -> Selector1/2, Compare To Constant/1
  Selector1/1 -> Switch1/1
  Switch1/1 -> Data Store Write/1
  Data Store Read2/1 -> Switch1/3
  Data Store Read1/1 -> Bitwise Operator2/1
  Constant2/1 -> Product/2, WarningByte/2

== system Ctrl_warning/Ctrl_warning_UpdateWarningStatus/UpdateWarningProperties/Payloadpdates ==
  "WarningID " : Inport
  WarningStatus : Inport  Port=2
  PayloadValue : Inport  Port=3
  ClearPayload : Subsystem  TreatAsAtomicUnit=on
      settings: RTWSystemCode=Inline
  Compare To Constant : simulink/Logic and Bit Operations/Compare To Constant  relop===  const=UI_WARNING_STATUS_OFF  OutDataTypeStr=boolean
  If : If  IfExpression=u1 ~= 0
  PayloadUpdate : Subsystem  TreatAsAtomicUnit=on
      settings: RTWSystemCode=Inline
  wires:
  PayloadValue/1 -> PayloadUpdate/2(Payload)
  "WarningID "/1 -> PayloadUpdate/1(WarningID), ClearPayload/1("WarningID ")
  If/2 -> PayloadUpdate/Action
  If/1 -> ClearPayload/Action
  Compare To Constant/1 -> If/1
  WarningStatus/1 -> Compare To Constant/1

== system Ctrl_warning/Ctrl_warning_UpdateWarningStatus/UpdateWarningProperties/EventUpdates/EventNone ==
  "WarningID " : Inport
  Action Port : ActionPort  ActionType=then
  Assignment : Assignment  IndexMode=Zero-based  DiagnosticForDimensions=Warning  IndexOptions=Index vector (port)  Indices=1  OutputSizes=14
  Bus Assignment : BusAssignment  AssignedSignals=ExtWarningCurrentEvent
  Constant : Constant  Value=UI_WARNING_EVENT_NONE  OutDataTypeStr=uint8
  Data Store Read : DataStoreRead  DataStoreName=l_ArbtnWarnData_S
  Data Store Read1 : DataStoreRead  DataStoreName=l_ArbtnWarnData_S
  Data Store Write : DataStoreWrite  DialogController=Simulink.DDGSource  DataStoreName=l_ArbtnWarnData_S
  Selector : Selector  IndexMode=Zero-based  IndexOptions=Index vector (port)  Indices=[1 3]  OutputSizes=1
  wires:
  Bus Assignment/1 -> Assignment/2
  Assignment/1 -> Data Store Write/1
  "WarningID "/1 -> Assignment/3, Selector/2
  Constant/1 -> Bus Assignment/2
  Data Store Read/1 -> Selector/1
  Selector/1 -> Bus Assignment/1
  Data Store Read1/1 -> Assignment/1

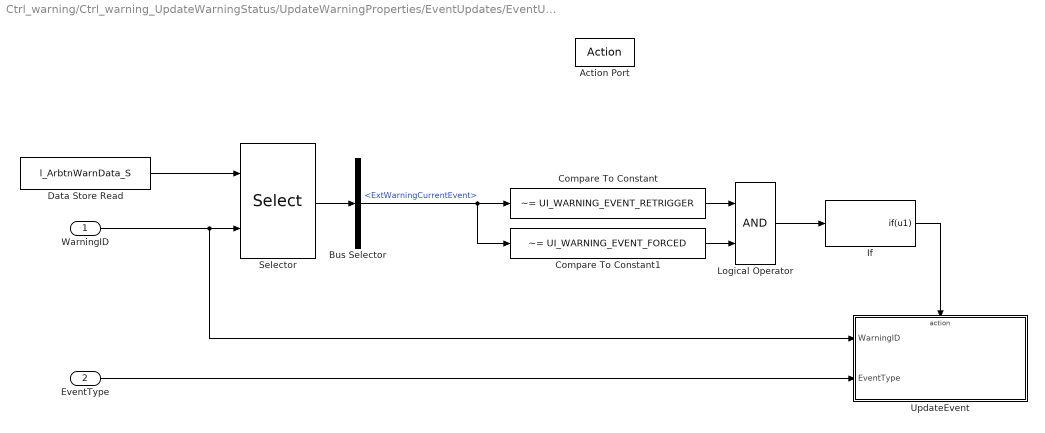
== system Ctrl_warning/Ctrl_warning_UpdateWarningStatus/UpdateWarningProperties/EventUpdates/EventUpdate ==
  WarningID : Inport
  EventType : Inport  Port=2
  Action Port : ActionPort  ActionType=else
  Bus Selector : BusSelector  OutputSignals=ExtWarningCurrentEvent
  Compare To Constant : simulink/Logic and Bit Operations/Compare To Constant  relop=~=  const=UI_WARNING_EVENT_RETRIGGER  OutDataTypeStr=boolean
  Compare To Constant1 : simulink/Logic and Bit Operations/Compare To Constant  relop=~=  const=UI_WARNING_EVENT_FORCED  OutDataTypeStr=boolean
  Data Store Read : DataStoreRead  DataStoreName=l_ArbtnWarnData_S
  If : If  IfExpression=u1  ShowElse=off
  Logical Operator : Logic  AllPortsSameDT=off  OutDataTypeStr=boolean
  Selector : Selector  IndexMode=Zero-based  IndexOptions=Index vector (port)  Indices=[1 3]  OutputSizes=1
  UpdateEvent : Subsystem  TreatAsAtomicUnit=on
  wires:
  Data Store Read/1 -> Selector/1
  Selector/1 -> Bus Selector/1
  Bus Selector/1 -> Compare To Constant/1, Compare To Constant1/1  "<ExtWarningCurrentEvent>"
  Compare To Constant/1 -> Logical Operator/1
  Compare To Constant1/1 -> Logical Operator/2
  Logical Operator/1 -> If/1
  If/1 -> UpdateEvent/Action
  EventType/1 -> UpdateEvent/2(EventType)
  WarningID/1 -> UpdateEvent/1("WarningID "), Selector/2

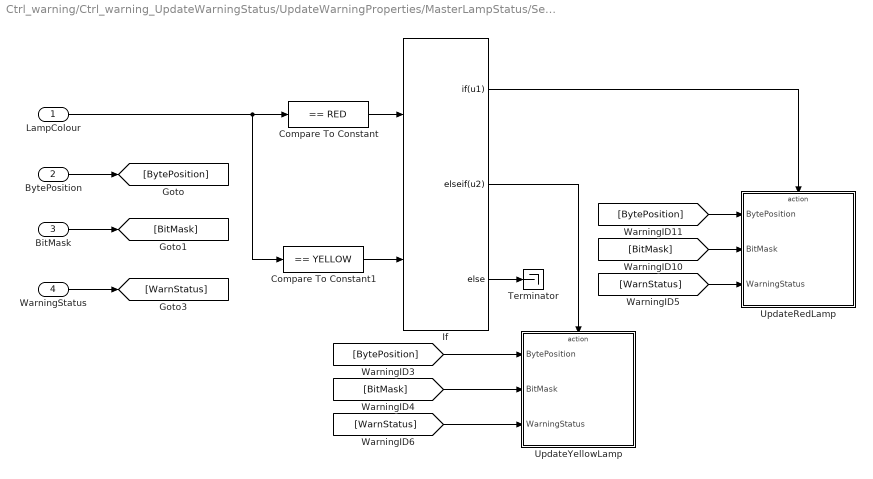
== system Ctrl_warning/Ctrl_warning_UpdateWarningStatus/UpdateWarningProperties/MasterLampStatus/SetMasterWarningLamp ==
  LampColour : Inport  OutDataTypeStr=uint8
  BytePosition : Inport  Port=2
  BitMask : Inport  Port=3
  WarningStatus : Inport  Port=4  OutDataTypeStr=uint8
  Compare To Constant : simulink/Logic and Bit Operations/Compare To Constant  relop===  const=RED  OutDataTypeStr=boolean
  Compare To Constant1 : simulink/Logic and Bit Operations/Compare To Constant  relop===  const=YELLOW  OutDataTypeStr=boolean
  If : If  NumInputs=2  IfExpression=u1  ElseIfExpressions=u2
  Terminator : Terminator
  UpdateRedLamp : Subsystem  TreatAsAtomicUnit=on
  UpdateYellowLamp : Subsystem  TreatAsAtomicUnit=on
  wires:
  BytePosition/1 -> [BytePosition]
  BitMask/1 -> [BitMask]
  Compare To Constant/1 -> If/1
  LampColour/1 -> Compare To Constant1/1, Compare To Constant/1
  [BytePosition] -> UpdateRedLamp/1(BytePosition)
  [BitMask] -> UpdateRedLamp/2(BitMask)
  Compare To Constant1/1 -> If/2
  [BytePosition] -> UpdateYellowLamp/1(BytePosition)
  [BitMask] -> UpdateYellowLamp/2(BitMask)
  WarningStatus/1 -> [WarnStatus]
  [WarnStatus] -> UpdateRedLamp/3(WarningStatus)
  [WarnStatus] -> UpdateYellowLamp/3(WarningStatus)
  If/1 -> UpdateRedLamp/Action
  If/3 -> Terminator/1
  If/2 -> UpdateYellowLamp/Action

== system Ctrl_warning/Ctrl_warning_UpdateWarningStatus/UpdateWarningProperties/Payloadpdates/ClearPayload ==
  "WarningID " : Inport
  Action Port : ActionPort  ActionType=then
  Assignment : Assignment  IndexMode=Zero-based  DiagnosticForDimensions=Warning  IndexOptions=Index vector (port)  Indices=1  OutputSizes=14
  Bus Assignment : BusAssignment  AssignedSignals=ExtWarningCurrentPayload
  Constant : Constant  Value=zeros(1,8)  OutDataTypeStr=PayloadArr_u8_8
  Data Store Read : DataStoreRead  DataStoreName=l_ArbtnWarnData_S
  Data Store Read1 : DataStoreRead  DataStoreName=l_ArbtnWarnData_S
  Data Store Write : DataStoreWrite  DialogController=Simulink.DDGSource  DataStoreName=l_ArbtnWarnData_S
  Selector : Selector  IndexMode=Zero-based  IndexOptions=Index vector (port)  Indices=[1 3]  OutputSizes=1
  wires:
  Data Store Read1/1 -> Assignment/1
  Selector/1 -> Bus Assignment/1
  Data Store Read/1 -> Selector/1
  Constant/1 -> Bus Assignment/2
  "WarningID "/1 -> Selector/2, Assignment/3
  Assignment/1 -> Data Store Write/1
  Bus Assignment/1 -> Assignment/2

== system Ctrl_warning/Ctrl_warning_UpdateWarningStatus/UpdateWarningProperties/Payloadpdates/PayloadUpdate ==
  WarningID : Inport
  Payload : Inport  Port=2
  Action Port : ActionPort  ActionType=else
  Compare To Constant2 : simulink/Logic and Bit Operations/Compare To Constant  relop=~=  const=EXTD_PAYLOAD_AVBLSTS  OutDataTypeStr=boolean
  Data Store Read : DataStoreRead  DataStoreName=l_ExtdPayoadCalld_u8
  If1 : If  IfExpression=u1  ShowElse=off
  Selector : Selector  IndexMode=Zero-based  IndexOptions=Index vector (port)  Indices=[1 3]  OutputSizes=1
  UpdateRecdPayload : Subsystem  TreatAsAtomicUnit=on
  wires:
  WarningID/1 -> UpdateRecdPayload/1("WarningID "), Selector/2
  Payload/1 -> UpdateRecdPayload/2(Payload)
  Compare To Constant2/1 -> If1/1
  Data Store Read/1 -> Selector/1
  Selector/1 -> Compare To Constant2/1
  If1/1 -> UpdateRecdPayload/Action

== system Ctrl_warning/Ctrl_warning_UpdateWarningStatus/UpdateWarningProperties/EventUpdates/EventUpdate/UpdateEvent ==
  "WarningID " : Inport
  EventType : Inport  Port=2
  Action Port : ActionPort  ActionType=then
  Assignment : Assignment  IndexMode=Zero-based  DiagnosticForDimensions=Warning  IndexOptions=Index vector (port)  Indices=1  OutputSizes=14
  Bus Assignment : BusAssignment  AssignedSignals=ExtWarningCurrentEvent
  Data Store Read : DataStoreRead  DataStoreName=l_ArbtnWarnData_S
  Data Store Read1 : DataStoreRead  DataStoreName=l_ArbtnWarnData_S
  Data Store Write : DataStoreWrite  DialogController=Simulink.DDGSource  DataStoreName=l_ArbtnWarnData_S
  Selector : Selector  IndexMode=Zero-based  IndexOptions=Index vector (port)  Indices=[1 3]  OutputSizes=1
  wires:
  Bus Assignment/1 -> Assignment/2
  Assignment/1 -> Data Store Write/1
  "WarningID "/1 -> Assignment/3, Selector/2
  Data Store Read/1 -> Selector/1
  Selector/1 -> Bus Assignment/1
  EventType/1 -> Bus Assignment/2
  Data Store Read1/1 -> Assignment/1

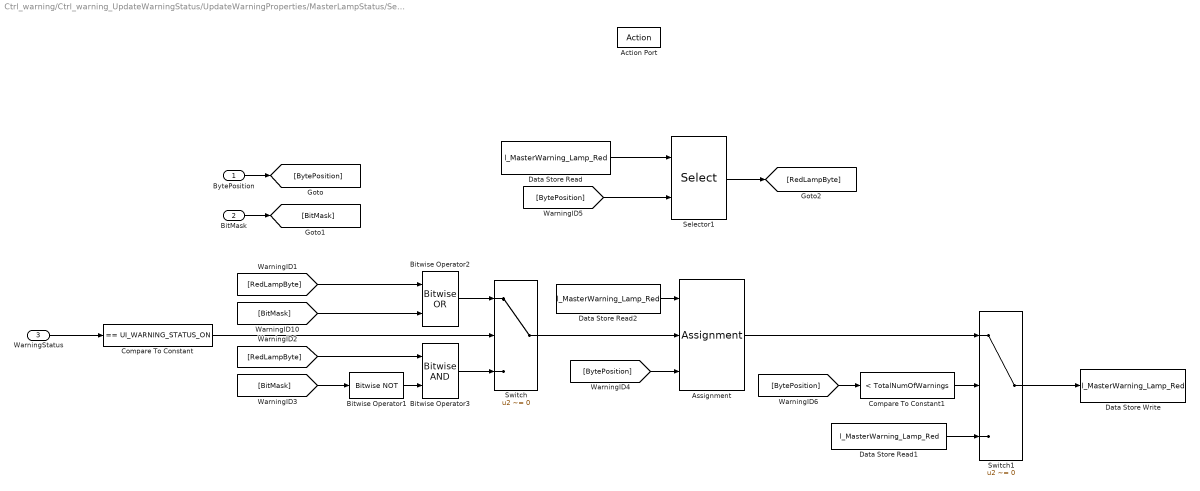
== system Ctrl_warning/Ctrl_warning_UpdateWarningStatus/UpdateWarningProperties/MasterLampStatus/SetMasterWarningLamp/UpdateRedLamp ==
  BytePosition : Inport
  BitMask : Inport  Port=2
  WarningStatus : Inport  Port=3  OutDataTypeStr=uint8
  Action Port : ActionPort  ActionType=then
  Assignment : Assignment  IndexMode=Zero-based  DiagnosticForDimensions=Warning  IndexOptions=Index vector (port)  Indices=1  OutputSizes=14
  Bitwise Operator1 : simulink/Logic and Bit Operations/Bitwise Operator  logicop=NOT  UseBitMask=off  BitMask=bin2dec('11011001')  BitMaskRealWorld=Stored Integer
  Bitwise Operator2 : simulink/Logic and Bit Operations/Bitwise Operator  logicop=OR  UseBitMask=off  NumInputPorts=2  BitMask=bin2dec('11011001')  BitMaskRealWorld=Stored Integer
  Bitwise Operator3 : simulink/Logic and Bit Operations/Bitwise Operator  logicop=AND  UseBitMask=off  NumInputPorts=2  BitMask=bin2dec('11011001')  BitMaskRealWorld=Stored Integer
  Compare To Constant : simulink/Logic and Bit Operations/Compare To Constant  relop===  const=UI_WARNING_STATUS_ON  OutDataTypeStr=boolean
  Compare To Constant1 : simulink/Logic and Bit Operations/Compare To Constant  relop=<  const=TotalNumOfWarnings  OutDataTypeStr=boolean
  Data Store Read : DataStoreRead  DataStoreName=l_MasterWarning_Lamp_Red
  Data Store Read1 : DataStoreRead  DataStoreName=l_MasterWarning_Lamp_Red
  Data Store Read2 : DataStoreRead  DataStoreName=l_MasterWarning_Lamp_Red
  Data Store Write : DataStoreWrite  DialogController=Simulink.DDGSource  DataStoreName=l_MasterWarning_Lamp_Red
  Selector1 : Selector  IndexMode=Zero-based  IndexOptions=Index vector (port)  Indices=[1 3]  OutputSizes=1
  Switch : Switch  Criteria=u2 ~= 0
  Switch1 : Switch  Criteria=u2 ~= 0
  wires:
  Data Store Read/1 -> Selector1/1
  WarningStatus/1 -> Compare To Constant/1
  BytePosition/1 -> [BytePosition]
  BitMask/1 -> [BitMask]
  [BitMask] -> Bitwise Operator2/2
  Compare To Constant/1 -> Switch/2
  Bitwise Operator2/1 -> Switch/1
  [RedLampByte] -> Bitwise Operator2/1
  [RedLampByte] -> Bitwise Operator3/1
  [BitMask] -> Bitwise Operator1/1
  Bitwise Operator1/1 -> Bitwise Operator3/2
  Bitwise Operator3/1 -> Switch/3
  Switch/1 -> Assignment/2
  [BytePosition] -> Assignment/3
  [BytePosition] -> Selector1/2
  [BytePosition] -> Compare To Constant1/1
  Selector1/1 -> [RedLampByte]
  Compare To Constant1/1 -> Switch1/2
  Switch1/1 -> Data Store Write/1
  Assignment/1 -> Switch1/1
  Data Store Read1/1 -> Switch1/3
  Data Store Read2/1 -> Assignment/1

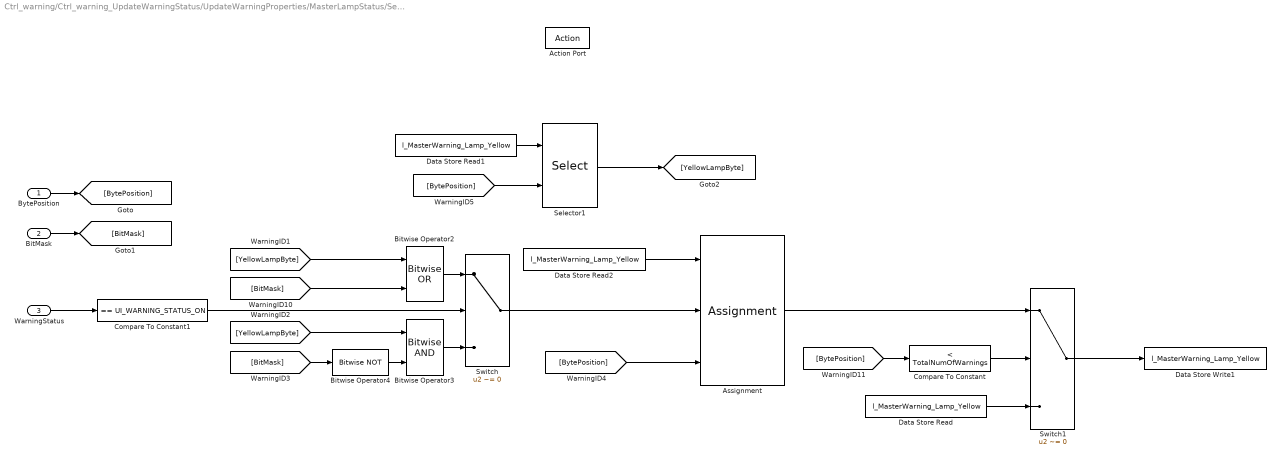
== system Ctrl_warning/Ctrl_warning_UpdateWarningStatus/UpdateWarningProperties/MasterLampStatus/SetMasterWarningLamp/UpdateYellowLamp ==
  BytePosition : Inport
  BitMask : Inport  Port=2
  WarningStatus : Inport  Port=3  OutDataTypeStr=uint8
  Action Port : ActionPort  ActionType=elseif
  Assignment : Assignment  IndexMode=Zero-based  DiagnosticForDimensions=Warning  IndexOptions=Index vector (port)  Indices=1  OutputSizes=14
  Bitwise Operator2 : simulink/Logic and Bit Operations/Bitwise Operator  logicop=OR  UseBitMask=off  NumInputPorts=2  BitMask=bin2dec('11011001')  BitMaskRealWorld=Stored Integer
  Bitwise Operator3 : simulink/Logic and Bit Operations/Bitwise Operator  logicop=AND  UseBitMask=off  NumInputPorts=2  BitMask=bin2dec('11011001')  BitMaskRealWorld=Stored Integer
  Bitwise Operator4 : simulink/Logic and Bit Operations/Bitwise Operator  logicop=NOT  UseBitMask=off  BitMask=bin2dec('11011001')  BitMaskRealWorld=Stored Integer
  Compare To Constant : simulink/Logic and Bit Operations/Compare To Constant  relop=<  const=TotalNumOfWarnings  OutDataTypeStr=boolean
  Compare To Constant1 : simulink/Logic and Bit Operations/Compare To Constant  relop===  const=UI_WARNING_STATUS_ON  OutDataTypeStr=boolean
  Data Store Read : DataStoreRead  DataStoreName=l_MasterWarning_Lamp_Yellow
  Data Store Read1 : DataStoreRead  DataStoreName=l_MasterWarning_Lamp_Yellow
  Data Store Read2 : DataStoreRead  DataStoreName=l_MasterWarning_Lamp_Yellow
  Data Store Write1 : DataStoreWrite  DialogController=Simulink.DDGSource  DataStoreName=l_MasterWarning_Lamp_Yellow
  Selector1 : Selector  IndexMode=Zero-based  IndexOptions=Index vector (port)  Indices=[1 3]  OutputSizes=1
  Switch : Switch  Criteria=u2 ~= 0
  Switch1 : Switch  Criteria=u2 ~= 0
  wires:
  [BytePosition] -> Assignment/3
  Switch/1 -> Assignment/2
  Bitwise Operator3/1 -> Switch/3
  Bitwise Operator4/1 -> Bitwise Operator3/2
  [BitMask] -> Bitwise Operator4/1
  [YellowLampByte] -> Bitwise Operator3/1
  [YellowLampByte] -> Bitwise Operator2/1
  Bitwise Operator2/1 -> Switch/1
  Compare To Constant1/1 -> Switch/2
  [BitMask] -> Bitwise Operator2/2
  BitMask/1 -> [BitMask]
  BytePosition/1 -> [BytePosition]
  WarningStatus/1 -> Compare To Constant1/1
  Data Store Read1/1 -> Selector1/1
  [BytePosition] -> Selector1/2
  [BytePosition] -> Compare To Constant/1
  Compare To Constant/1 -> Switch1/2
  Selector1/1 -> [YellowLampByte]
  Assignment/1 -> Switch1/1
  Switch1/1 -> Data Store Write1/1
  Data Store Read/1 -> Switch1/3
  Data Store Read2/1 -> Assignment/1

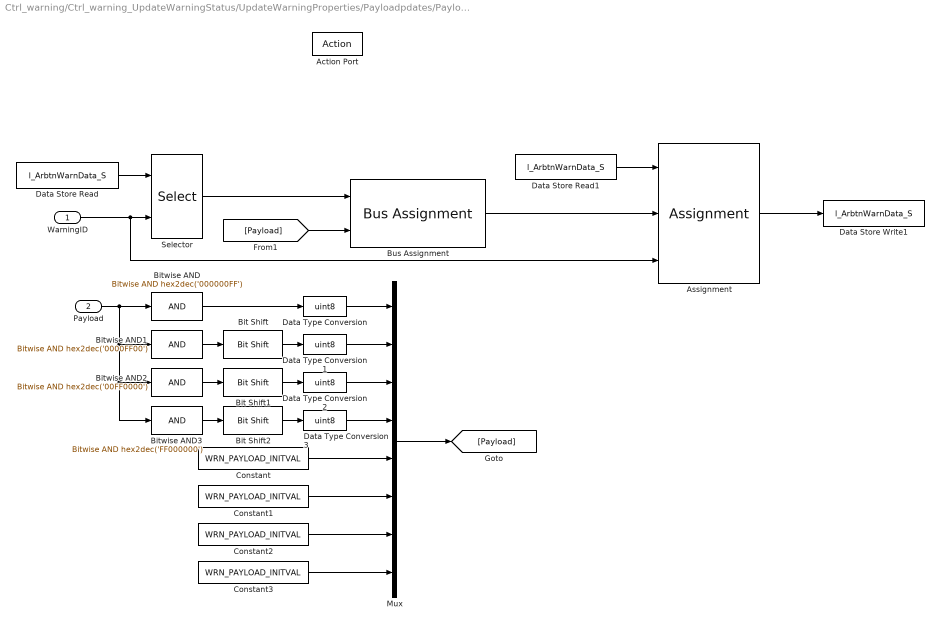
== system Ctrl_warning/Ctrl_warning_UpdateWarningStatus/UpdateWarningProperties/Payloadpdates/PayloadUpdate/UpdateRecdPayload ==
  "WarningID " : Inport
  Payload : Inport  Port=2
  Action Port : ActionPort  ActionType=then
  Assignment : Assignment  IndexMode=Zero-based  DiagnosticForDimensions=Warning  IndexOptions=Index vector (port)  Indices=1  OutputSizes=14
  Bit Shift : hdlsllib/Logic and Bit Operations/Bit Shift  mode=Shift Right Logical  N=8
      settings: SourceProductName=HDL Coder  SourceProductBaseCode=HD
  Bit Shift1 : hdlsllib/Logic and Bit Operations/Bit Shift  mode=Shift Right Logical  N=16
      settings: SourceProductName=HDL Coder  SourceProductBaseCode=HD
  Bit Shift2 : hdlsllib/Logic and Bit Operations/Bit Shift  mode=Shift Right Logical  N=24
      settings: SourceProductName=HDL Coder  SourceProductBaseCode=HD
  Bitwise AND : simulink/Logic and Bit Operations/Bitwise Operator  logicop=AND  UseBitMask=on  BitMask=hex2dec('000000FF')  BitMaskRealWorld=Stored Integer
  Bitwise AND1 : simulink/Logic and Bit Operations/Bitwise Operator  logicop=AND  UseBitMask=on  BitMask=hex2dec('0000FF00')  BitMaskRealWorld=Stored Integer
  Bitwise AND2 : simulink/Logic and Bit Operations/Bitwise Operator  logicop=AND  UseBitMask=on  BitMask=hex2dec('00FF0000')  BitMaskRealWorld=Stored Integer
  Bitwise AND3 : simulink/Logic and Bit Operations/Bitwise Operator  logicop=AND  UseBitMask=on  BitMask=hex2dec('FF000000')  BitMaskRealWorld=Stored Integer
  Bus Assignment : BusAssignment  AssignedSignals=ExtWarningCurrentPayload
  Constant{,1..3} (4 alike) : Constant  Value=WRN_PAYLOAD_INITVAL
  Data Store Read : DataStoreRead  DataStoreName=l_ArbtnWarnData_S
  Data Store Read1 : DataStoreRead  DataStoreName=l_ArbtnWarnData_S
  Data Store Write1 : DataStoreWrite  DataStoreName=l_ArbtnWarnData_S
  Data Type Conversion{,1..3} (4 alike) : DataTypeConversion  OutDataTypeStr=uint8
  Mux : Mux  Inputs=8
  Selector : Selector  IndexMode=Zero-based  IndexOptions=Index vector (port)  Indices=[1 3]  OutputSizes=1
  wires:
  Bus Assignment/1 -> Assignment/2
  Assignment/1 -> Data Store Write1/1
  "WarningID "/1 -> Assignment/3, Selector/2
  Data Store Read/1 -> Selector/1
  Selector/1 -> Bus Assignment/1
  Data Store Read1/1 -> Assignment/1
  Payload/1 -> Bitwise AND2/1, Bitwise AND3/1, Bitwise AND1/1, Bitwise AND/1
  Bitwise AND/1 -> Data Type Conversion/1
  Mux/1 -> [Payload]
  [Payload] -> Bus Assignment/2
  Data Type Conversion/1 -> Mux/1
  Data Type Conversion1/1 -> Mux/2
  Data Type Conversion2/1 -> Mux/3
  Data Type Conversion3/1 -> Mux/4
  Bit Shift/1 -> Data Type Conversion1/1
  Bitwise AND1/1 -> Bit Shift/1
  Bit Shift1/1 -> Data Type Conversion2/1
  Bitwise AND2/1 -> Bit Shift1/1
  Bitwise AND3/1 -> Bit Shift2/1
  Bit Shift2/1 -> Data Type Conversion3/1
  Constant/1 -> Mux/5
  Constant1/1 -> Mux/6
  Constant2/1 -> Mux/7
  Constant3/1 -> Mux/8

== stateflow chart Ctrl_warning/Ctrl_warning_Get_Red_MasterLamp_Status/Chart ==
  state LampStatus [function]
    (default) -> (junction 38)
    (junction 38) -> (junction 33) [order 1] : [(l_MasterWarning_Lamp_Red[fl_RedLampIdx_u16] != uint8(0))]
    (junction 33) -> (junction 37) : {
        | fl_RedLampSts_u8 = uint8(1);
        | }
    (junction 38) -> (junction 36) [order 2]
    (junction 37) -> (junction 36)
  (default) -> (junction 20) : /* Master warning Lamp Status */
      | { fl_RedLampSts_u8 = uint8(0);}
  (junction 20) -> (junction 21) : {fl_RedLampIdx_u16 = uint16(0);}
  (junction 21) -> (junction 19) [order 1] : [fl_RedLampIdx_u16 < TotalNumOfWarnings]
  (junction 22) -> (junction 21) : {fl_RedLampIdx_u16 = fl_RedLampIdx_u16 + ...
      |  uint16(1);}
  (junction 21) -> (junction 23) [order 2]
  (junction 19) -> (junction 22) : {LampStatus();}
  data: l_MasterWarning_Lamp_Red data_store_memory; fl_RedLampIdx_u16 local uint16 =0; fl_RedLampSts_u8 output uint8; TotalNumOfWarnings parameter

== stateflow chart Ctrl_warning/Ctrl_warning_Get_Yellow_MasterLamp_Status/Chart ==
  state LampStatus [function]
    (default) -> (junction 38)
    (junction 38) -> (junction 33) [order 1] : [(l_MasterWarning_Lamp_Yellow[fl_YellowLampIdx_u16] != 0)]
    (junction 33) -> (junction 37) : {
        | fl_YellowLampSts_u8 = uint8(1);
        | }
    (junction 38) -> (junction 36) [order 2]
    (junction 37) -> (junction 36)
  (default) -> (junction 20) : /* Master warning Lamp Status */
      | { fl_YellowLampSts_u8 = uint8(0);}
  (junction 20) -> (junction 21) : {fl_YellowLampIdx_u16 = uint16(0);}
  (junction 21) -> (junction 19) [order 1] : [fl_YellowLampIdx_u16 < TotalNumOfWarnings]
  (junction 22) -> (junction 21) : {fl_YellowLampIdx_u16 = fl_YellowLampIdx_u16 ...
      | + uint16(1);}
  (junction 21) -> (junction 23) [order 2]
  (junction 19) -> (junction 22) : {LampStatus();}
  data: l_MasterWarning_Lamp_Yellow data_store_memory; fl_YellowLampIdx_u16 local uint16 =0; fl_YellowLampSts_u8 output uint8; TotalNumOfWarnings parameter
